simulink model "tutorial2"  (Simulink 2.20)
settings: Solver=ode5  StartTime=0.0  StopTime=tstop  FixedStep=tstep  MaxStep=tstep  RelTol=1e-3  AbsTol=1e-3
settings Model: SaveTime=off  SaveOutput=off  ConsistencyChecking=off  RTWPlaceOutputsASAP=off

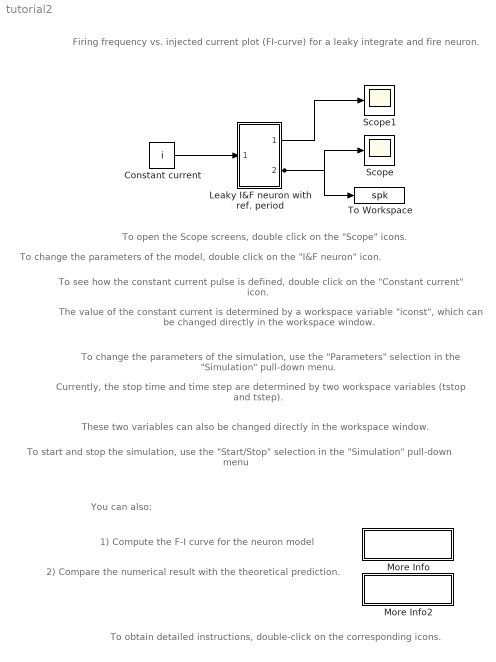
== system tutorial2 ==
  note: To open the Scope screens, double click on the "Scope" icons.
  note: Firing frequency vs. injected current plot (FI-curve) for a leaky
      | integrate and fire neuron.
  note: To change the parameters of the model,
      | double click on the "I&F neuron" icon.
  note: To see how the constant current pulse is defined, double click
      | on the "Constant current" icon.
  note: Currently, the stop time and time step are determined by two
      | workspace variables (tstop and tstep).
  note: To change the parameters of the simulation, use the "Parameters"
      | selection in the "Simulation" pull-down menu.
  note: The value of the constant current is determined by a workspace
      | variable "iconst", which can be changed directly in the workspace
      | window.
  note: These two variables can also be changed directly in the
      | workspace window.
  note: To start and stop the simulation, use the "Start/Stop"
      | selection in the "Simulation" pull-down menu
  note: You can also:
  note: 1) Compute the F-I curve for the neuron model
  note: 2) Compare the numerical result with the
      | theoretical prediction.
  note: To obtain detailed instructions, double-click on the corresponding
      | icons.
  Constant current : Constant  Value=i  mask(constant current){@1=iconst}
      mask prompts: @1 "constant current value [nA]"
      mask help: Parameter
      mask init:
      | i = @1;
      mask Help: Provides a constant input current
  Leaky I&F neuron with ref. period : Subsystem  mask(L I&F ref. per.){@1=tstep, @2=10, @3=.5, @4=50, @5=5}
      mask prompts: @1 "time step [msec]"; @2 "threshold [mV]"; @3 "Capacitance [nF]"; @4 "Resistance [MOhms]"; @5 "refractory period [msec]"
      mask help: Parameters
      mask init:
      | dt = @1; thres = @2; C = @3; R = @4; ref = @5;
      mask Help: For a detailled description of the model, please type 'help liandfr' in the main matlab window.
      mask Display: disp('Vm \n\n spikes')
  More Info : Subsystem
      mask Display: disp('Numerical\nFI-curve')
  More Info2 : Subsystem
      mask Display: disp('Theoretical\nFI-curve')
  Scope : Scope
      settings: TickLabels=on  TimeRange=500.000000  YMin=-2.000000  YMax=2.000000  SaveToWorkspace=off  SaveName=ScopeData
  Scope1 : Scope
      settings: TickLabels=on  TimeRange=500.000000  YMin=-15.000000  YMax=15.000000  SaveToWorkspace=off  SaveName=ScopeData
  To Workspace : ToWorkspace  VariableName=spk  SampleTime=0
      settings: Buffer=ceil(tstop/tstep)
  wires:
  Constant current/1 -> Leaky I&F neuron with ref. period/1(in_1)
  Leaky I&F neuron with ref. period/2(out_1) -> Scope/1, To Workspace/1
  Leaky I&F neuron with ref. period/1(out_2) -> Scope1/1

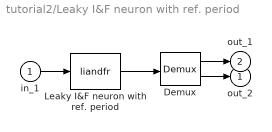
== system tutorial2/Leaky I&F neuron with ref. period ==
  in_1 : Inport  Port=1  PortWidth=-1  SampleTime=-1
  Demux : Demux  Outputs=2
  Leaky I&F neuron with ref. period : S-Function  FunctionName=liandfr  Parameters=dt,thres,C,R,ref  PortCounts=[]  SFunctionModules=''
  out_2 : Outport  Port=1  InitialOutput=0
  out_1 : Outport  Port=2  InitialOutput=0
  wires:
  Leaky I&F neuron with ref. period/1 -> Demux/1
  Demux/1 -> out_1/1
  Demux/2 -> out_2/1
  in_1/1 -> Leaky I&F neuron with ref. period/1

== system tutorial2/More Info ==
  note: To compute the FI-curve of the model, follow the
      | steps described below:
  note: 1) Call the ficurve script by entering:
  note: ficurve
  note: in the workspace window.
  note: 2) The first time that "ficurve" is called, it will ask for :
  note: -the name of the model (answer: tutorial2),
  note: -the name of the variable containing
      | the spike train (answer: spk)
  note: -the name of the input parameter
      | to be varied (answer: iconst),
  note: -a vector of values to be used for "iconst"
      | in the simulations (answer: [0:0.2:4]).
  note: For subsequent calls, ficurve will use the same
      | values for all the variables entered in step 2).
  note: It is possible to test new values of iconst by
      | updating the vector of values (see 2) above). Enter:
  note: values = [i_min:i_step:i_max];
  note: in the workspace window, where i_min, i_step and i_max
      | are the minimal, step increment and maximal value of
      | the current, respectively. Then call the script ficurve again,
      | as in 1).
  note: The effects of changing other model parameters can
      | be studied in a similar way, by changing the name
      | of the parameter to be varied and/or by modifying the
      | "ficurve" script.

== system tutorial2/More Info2 ==
  note: The parameters are:
  note: in the workspace window.
  note: 0.5 = Capacity of the model cell (nF)
  note: 10 = spike threshold (mV)
  note: 50 = resistance of the model cell (MOhms).
  note: 5 = refractory period (msec)
  note: val = vector of current values
  note: To compare the theoretical FI-curve with the
      | previously obtained numerical FI-curve, enter
  note: hold on
  note: fithlifref(10,0.5,50,5,values).
